simulink model "temperal_logic"  (R2019a)
settings: Solver=FixedStepDiscrete  StartTime=0.0  StopTime=50  FixedStep=0.5  RelTol=1e-3
settings Model: Creator=admin  LastModifiedBy=admin

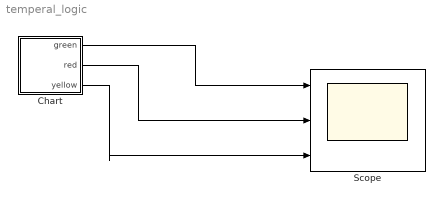
== system temperal_logic ==
  Chart : Stateflow chart  BlockKeywords=__PRM__SERIALIZED__DATA__:Stateflow Chart,Stateflow Diagram  TreatAsAtomicUnit=on
  Scope : Scope  NumInputPorts=3
  wires:
  Chart/1(green) -> Scope/1
  Chart/2(red) -> Scope/2
  Chart/3(yellow) -> Scope/3

== stateflow chart temperal_logic/Chart ==
  state go1
    en:green=1;
    ex:green=0
  state go [commented out]
    en:green=1;
    ex:green=0
  state preparetostop1
    en:yellow=1;
    ex:yellow=0;
  state preparetostop [commented out]
    en:yellow=1;
    ex:yellow=0;
  state red1
    en:red=1;
    ex:red=0;
  state red [commented out]
    en:red=1;
    ex:red=0;
  (default) -> go1
  (default) -> go [commented out]
  red1 -> go1
  red -> go [commented out]
  go1 -> preparetostop1 : after(5,tick)
  go -> preparetostop [commented out] : after(5,sec)
  preparetostop1 -> red1 : after(5,tick)
  preparetostop -> red [commented out] : after(5,sec)
  data: green output; red output; yellow output
